simulink model "part10"  (R2021b)
settings: Solver=ode5  StartTime=0.0  StopTime=5  FixedStep=1e-3  MaxStep=0.001  RelTol=1e-3  AbsTol=1e-5
model workspace (MATLAB code in the model file):
  | Ts=1e-3;
values from neighbouring files (symbols this model uses):
  m = 100 + a    (= 105)    [const.m]
libraries: vrlib x2
Description:
  | Magnetic Levitation Model
  | 
  | vrmaglev is an example showing the interaction between dynamic models in Simulink(R)
  | and virtual worlds. The Simulink model represents the HUMUSOFT(R) CE152 Magnetic Levitation
  | educational / presentation scale model. (http://www.humusoft.com/link/models)
  | 
  | The plant model is controlled by a PID controller with feed forward to cope with the nonlinearity
  | of the magnetic levitation system.
  | 
  | The position of the ball responds to the changing value of the setpoint. You can observe
  | this change not only in the Scope window, but also in a viewer window displaying
  | the virtual world. Note that the position of the ball represents the real dynamics of the system.
  | If you switch the VRML viewer to the Camera 3 viewpoint, you can observe and control the ball easier.
  | 
  | There are two possible methods of setting the ball position setpoint - using a Signal Generator
  | and visually by clicking at a desired position in the virtual reality scene.
  | 
  | In the virtual scene, a VRML sensor is defined. If you click in the space between the magnetic coil
  | and the bottom plate, VRML sensor is updated and its value is read into Simulink model using the
  | VR Source block.
settings Model: FPTRunName=Active  ExtModeTrigDuration=5000  ExtModeTrigLevel=0.500000  Creator=The MathWorks, Inc.  LastModifiedBy=aaomi
settings SolverCC: AutoScaleAbsTol=off  AlgebraicLoopSolver=TrustRegion
settings DataIOCC: SaveFormat=Array  SaveOutput=off  SaveTime=off  ReturnWorkspaceOutputs=off  SignalLoggingName=logsOut
settings OptimizationCC: BlockReduction=off  BooleanDataType=off  OptimizeBlockIOStorage=off  BufferReuse=off  GlobalBufferReuse=off  ExpressionFolding=off  ExpressionDepthLimit=2147483647  LocalBlockOutputs=off  InitFltsAndDblsToZero=on  LifeSpan=inf
settings DebuggingCC: UnderspecifiedInitializationDetection=Classic  MergeDetectMultiDrivingBlocksExec=none  CheckExecutionContextPreStartOutputMsg=on  SignalResolutionControl=TryResolveAllWithWarning  MultiTaskDSMMsg=warning  MultiTaskCondExecSysMsg=none  FcnCallInpInsideContextMsg=warning  StateNameClashWarn=warning  SFUnexpectedBacktrackingDiag=warning  SFNoUnconditionalDefaultTransitionDiag=warning  SFExecutionAtInitializationDiag=none  SFMachineParentedDataDiag=warning  ArithmeticOperatorsInVariantConditions=warning
settings HardwareCC: ProdBitPerPointer=32  ProdBitPerSizeT=32  ProdBitPerPtrDiffT=32  ProdLargestAtomicFloat=None  ProdIntDivRoundTo=Undefined  ProdEndianess=Unspecified  ProdWordSize=32  ProdHWDeviceType=32-bit Generic  TargetUnknown=on
settings ModelReferenceCC: UpdateModelReferenceTargets=IfOutOfDate  PropagateSignalLabelsOutOfModel=off
settings SFSimCC: SimUseLocalCustomCode=off  CustomCodeUndefinedFunction=UseInterfaceOnly
settings RTWCC: RetainRTWFile=on  RTWUseLocalCustomCode=off
settings CodeAppCC: StateflowObjectComments=on
settings GRTTargetCC: TargetFcnLib=ansi_tfl_tmw.mat  TargetLangStandard=C89/C90 (ANSI)  CombineOutputUpdateFcns=off  GRTInterface=on
settings ConfigComp: CovMetricSettings=d  CovSaveCumulativeToWorkspaceVar=on  CovSaveSingleToWorkspaceVar=on  CovExternalEMLEnable=off  CovSFcnEnable=off

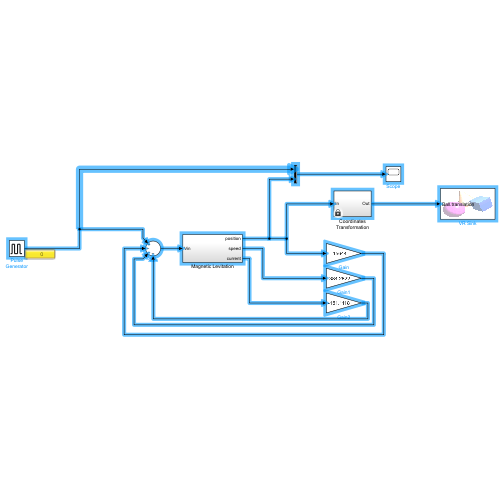
[thumbnail: Simulink's stored preview of the top-level diagram]
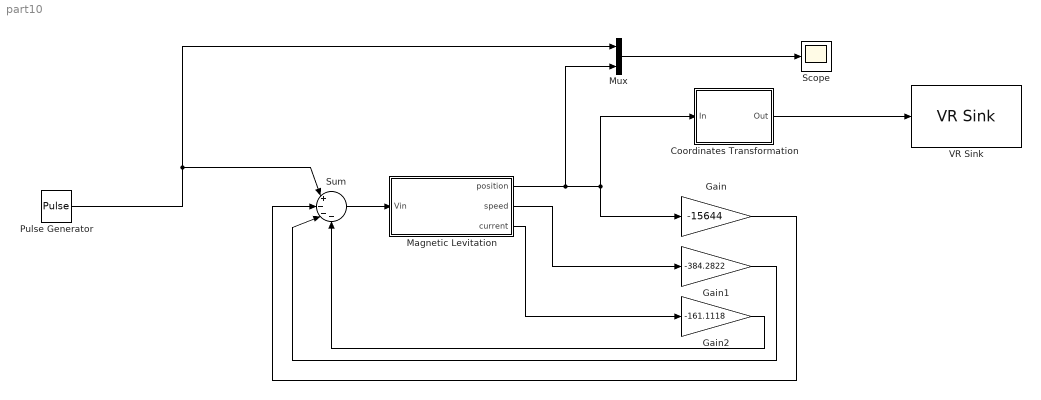
== system part10 ==
  Coordinates Transformation : Subsystem
  Gain : Gain  Gain=-15644
  Gain1 : Gain  Gain=-384.2822
  Gain2 : Gain  Gain=-161.1118
  Magnetic Levitation : Subsystem
  Mux : Mux  Inputs=2
  Pulse Generator : DiscretePulseGenerator  PulseType=Time based  Period=10  PulseWidth=50
  Scope : Scope
  Sum : Sum  Inputs=|+---  InputSameDT=on  SaturateOnIntegerOverflow=on  OutDataTypeStr=Inherit: Same as first input
  VR Sink : vrlib/VR Sink  InstantiateOnLoad=on  SampleTime=0.02  ViewEnable=on  RemoteChange=off  RemoteView=off  FieldsWritten=Ball.translation.3.1.1.double  WorldFileName=maglev.wrl  WorldDescription=VR Magnetic Levitation Model  AutoView=on  VideoDimensions=[]  AllowVariableSize=off  FigureProperties="{'Position', 'Name', 'Viewpoint', 'CameraBound', 'CameraDirection', 'CameraPosition', 'CameraUpVector', 'ZoomFactor', 'Antialiasing', 'Headlight', 'Lighting', 'NavPanel', 'Sound', 'StatusBar', 'Stereo3D', 'Stereo3DCameraOffset', 'Stereo3DHIT', 'ToolBar', 'Textures', 'Transparency', 'Triad', 'Wireframe', 'NavZones', 'NavMode', 'NavSpeed', 'CaptureFileFormat', 'CaptureFileName', 'Record2DCompressMethod', 'Record2DCompressQuality', 'Record2D', 'Record2DFileName', 'Record2DFPS'; [5.0000000000000000e+00   9.2000000000000000e+01   5.7600000000000000e+02   3.5000000000000000e+02], 'VR Magnetic Levitation Model', 'Camera 1', 'on', [0.0000000000000000e+00   0.0000000000000000e+00  -1.0000000000000000e+00], [0.0000000000000000e+00   0.0000000000000000e+00   0.0000000000000000e+00], [0.0000000000000000e+00   1.0000000000000000e+00   0.0000000000000000e+00], [1.0000000000000000e+00], 'on', 'off', 'on', 'halfbar', 'on', 'on', 'off', [1.0000000149011612e-01], [0.0000000000000000e+00], 'on', 'on', 'on', 'none', 'off', 'off', 'examine', 'normal', 'tif', '%f_anim_%n.tif', 'auto', [7.5000000000000000e+01], 'off', '%f_anim_%n.avi', 'auto'}"
  wires:
  Mux/1 -> Scope/1
  Coordinates Transformation/1(Out) -> VR Sink/1
  Magnetic Levitation/1(position) -> Gain/1, Coordinates Transformation/1(In), Mux/2
  Sum/1 -> Magnetic Levitation/1(Vin)
  Pulse Generator/1 -> Sum/1, Mux/1
  Magnetic Levitation/2(speed) -> Gain1/1
  Magnetic Levitation/3(current) -> Gain2/1
  Gain2/1 -> Sum/4
  Gain1/1 -> Sum/3
  Gain/1 -> Sum/2

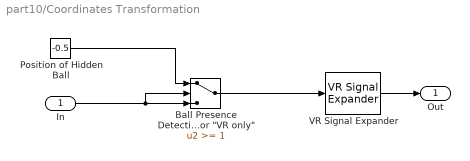
== system part10/Coordinates Transformation ==
  In : Inport
  "Ball Presence Detection Value > Threshold = Ball Not Present 1 for \"VR only\"" : Switch  Threshold=1  InputSameDT=on
  Position of Hidden Ball : Constant  Value=-0.5
  VR Signal Expander : vrlib/VR Signal Expander  outwidth=3  outidx=[2]
  Out : Outport
  wires:
  Position of Hidden Ball/1 -> "Ball Presence Detection Value > Threshold = Ball Not Present 1 for \"VR only\""/1
  In/1 -> "Ball Presence Detection Value > Threshold = Ball Not Present 1 for \"VR only\""/3, "Ball Presence Detection Value > Threshold = Ball Not Present 1 for \"VR only\""/2
  "Ball Presence Detection Value > Threshold = Ball Not Present 1 for \"VR only\""/1 -> VR Signal Expander/1
  VR Signal Expander/1 -> Out/1

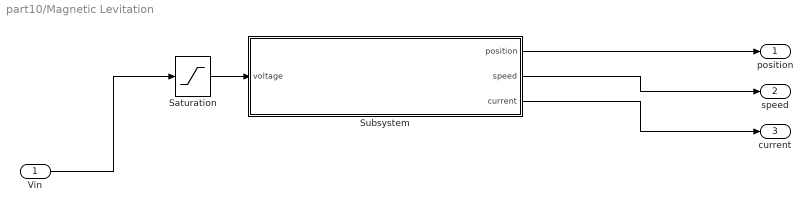
== system part10/Magnetic Levitation ==
  Vin : Inport
  Saturation : Saturate  UpperLimit=10  LowerLimit=0  ZeroCross=off
  Subsystem : Subsystem
  position : Outport
  speed : Outport  Port=2
  current : Outport  Port=3
  wires:
  Vin/1 -> Saturation/1
  Saturation/1 -> Subsystem/1(voltage)
  Subsystem/1("position ") -> position/1
  Subsystem/2(speed) -> speed/1
  Subsystem/3(current) -> current/1

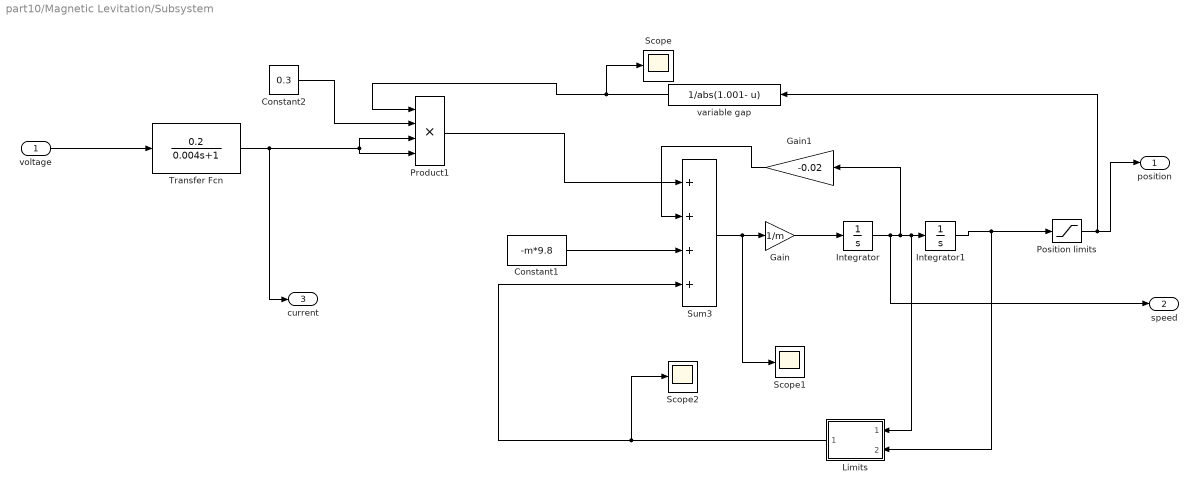
== system part10/Magnetic Levitation/Subsystem ==
  voltage : Inport
  Constant1 : Constant  Value=-m*9.8
  Constant2 : Constant  Value=0.3
  Gain : Gain  Gain=1/m
  Gain1 : Gain  Gain=-0.02
  Integrator : Integrator
  Integrator1 : Integrator  LimitOutput=on  UpperSaturationLimit=1  LowerSaturationLimit=0
  Limits : Subsystem
      mask Display: disp('LIMIT')
  Position limits : Saturate  UpperLimit=0.998  LowerLimit=0.001  ZeroCross=off
  Product1 : Product  Inputs=4
  Scope : Scope
  Scope1 : Scope
  Scope2 : Scope
  Sum3 : Sum  Inputs=++++
  Transfer Fcn : TransferFcn  Numerator=[0.2]  Denominator=[0.004 1]
  variable gap : Fcn  Expr=1/abs(1.001- u)
  "position " : Outport
  speed : Outport  Port=2
  current : Outport  Port=3
  wires:
  Position limits/1 -> variable gap/1, "position "/1
  Integrator1/1 -> Limits/2(position), Position limits/1
  Sum3/1 -> Scope1/1, Gain/1
  Constant2/1 -> Product1/2
  Constant1/1 -> Sum3/3
  variable gap/1 -> Scope/1, Product1/1
  Gain1/1 -> Sum3/2
  Gain/1 -> Integrator/1
  Integrator/1 -> speed/1, Limits/1(velocity), Integrator1/1, Gain1/1
  Product1/1 -> Sum3/1
  Transfer Fcn/1 -> current/1, Product1/3, Product1/4
  voltage/1 -> Transfer Fcn/1
  Limits/1(force) -> Scope2/1, Sum3/4

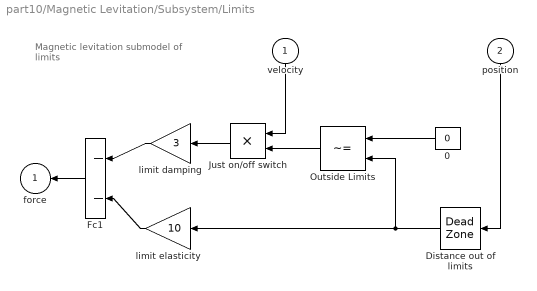
== system part10/Magnetic Levitation/Subsystem/Limits ==
  note: Magnetic levitation
      | submodel of limits
  velocity : Inport
  position : Inport  Port=2
  0 : Constant  Value=0
  Distance out of limits : DeadZone  LowerValue=0.002  UpperValue=1  ZeroCross=off  SaturateOnIntegerOverflow=on
  Fc1 : Sum  Inputs=--  InputSameDT=on  SaturateOnIntegerOverflow=on  OutDataTypeStr=Inherit: Same as first input
  "Just on/off switch " : Product  InputSameDT=on  SaturateOnIntegerOverflow=on  OutDataTypeStr=Inherit: Same as first input
  Outside Limits : RelationalOperator  Operator=~=  RndMeth=Nearest  InputSameDT=on
  limit damping : Gain  Gain=3  SaturateOnIntegerOverflow=on  OutDataTypeStr=Inherit: Same as input  ParamDataTypeStr=Inherit: Same as input
  limit elasticity : Gain  Gain=10  SaturateOnIntegerOverflow=on  OutDataTypeStr=Inherit: Same as input  ParamDataTypeStr=Inherit: Same as input
  force : Outport
  wires:
  Distance out of limits/1 -> Outside Limits/2, limit elasticity/1
  limit damping/1 -> Fc1/1
  limit elasticity/1 -> Fc1/2
  Outside Limits/1 -> "Just on/off switch "/2
  0/1 -> Outside Limits/1
  "Just on/off switch "/1 -> limit damping/1
  velocity/1 -> "Just on/off switch "/1
  Fc1/1 -> force/1
  position/1 -> Distance out of limits/1
